simulink model "verify_Storage_Type_1_mdl"  (R2018b)
settings: Solver=ode45  StartTime=time(1)  StopTime=time(end)  MaxStep=time(2)-time(1)  RelTol=1e-3  EnableMultiTasking=on
libraries: carnot x12
settings Model: DEBUGGLOBALLEVEL=DEBUGLEVEL  DEBUGMAXTOTALWARNINGS=0  DEBUGMAXCONSECUTIVEWARNINGS=0  DEBUGWRITETOFILE=0  DEBUGFILENAME='error.txt'  Creator=drhf  LastModifiedBy=P41573
settings DataIOCC: SaveFormat=Array  SignalLoggingSaveFormat=ModelDataLogs
settings OptimizationCC: ExpressionDepthLimit=2147483647  LifeSpan=inf
settings DebuggingCC: UnderspecifiedInitializationDetection=Classic  MergeDetectMultiDrivingBlocksExec=none  SolverPrmCheckMsg=warning  FcnCallInpInsideContextMsg=warning  StateNameClashWarn=warning  SFUnexpectedBacktrackingDiag=warning  SFNoUnconditionalDefaultTransitionDiag=warning  SFExecutionAtInitializationDiag=none
settings HardwareCC: ProdBitPerPointer=32  ProdBitPerSizeT=32  ProdBitPerPtrDiffT=32  ProdLargestAtomicFloat=None  ProdIntDivRoundTo=Undefined  ProdEndianess=Unspecified  ProdWordSize=32  ProdHWDeviceType=32-bit Generic
settings ModelReferenceCC: PropagateSignalLabelsOutOfModel=off
settings SFSimCC: SimUseLocalCustomCode=off
settings RTWCC: RTWUseLocalCustomCode=off
settings CodeAppCC: StateflowObjectComments=on
settings GRTTargetCC: TargetLangStandard=C89/C90 (ANSI)  GeneratePreprocessorConditionals=Disable all  CombineOutputUpdateFcns=off  GRTInterface=on
settings ConfigComp: CovMetricSettings=dw  CovHtmlReporting=on  CovSaveCumulativeToWorkspaceVar=on  CovSaveSingleToWorkspaceVar=on  CovExternalEMLEnable=off

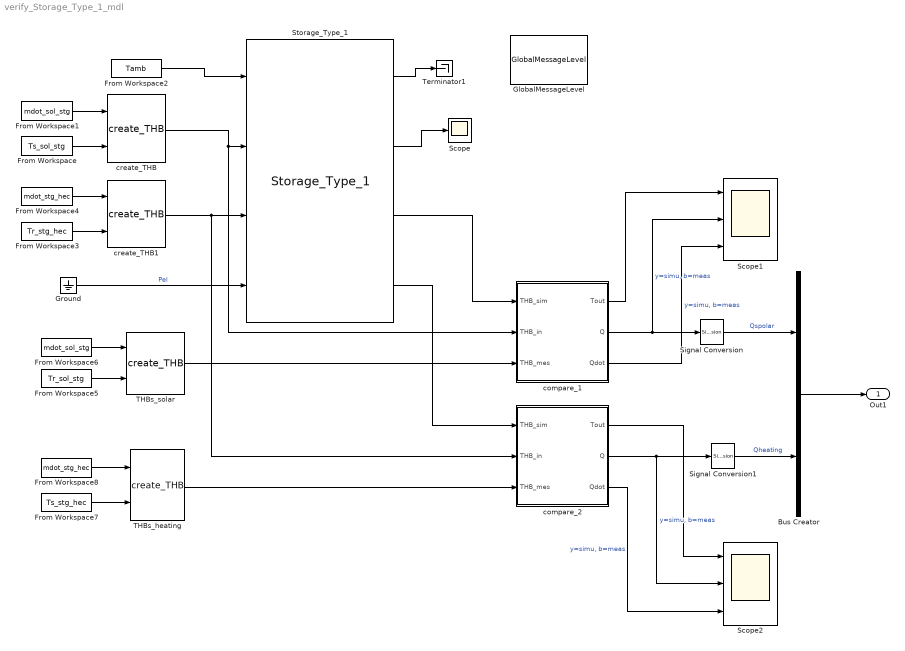
== system verify_Storage_Type_1_mdl ==
  Bus Creator : BusCreator  Inputs=2
  From Workspace : FromWorkspace  VariableName=Ts_sol_stg  SampleTime=0
  From Workspace1 : FromWorkspace  VariableName=mdot_sol_stg  SampleTime=0
  From Workspace2 : FromWorkspace  VariableName=Tamb  SampleTime=0
  From Workspace3 : FromWorkspace  VariableName=Tr_stg_hec  SampleTime=0
  From Workspace4 : FromWorkspace  VariableName=mdot_stg_hec  SampleTime=0
  From Workspace5 : FromWorkspace  VariableName=Tr_sol_stg  SampleTime=0
  From Workspace6 : FromWorkspace  VariableName=mdot_sol_stg  SampleTime=0
  From Workspace7 : FromWorkspace  VariableName=Ts_stg_hec  SampleTime=0
  From Workspace8 : FromWorkspace  VariableName=mdot_stg_hec  SampleTime=0
  GlobalMessageLevel : carnot/Toolbox/GlobalMessageLevel  GLOBALLOCAL=global  DEBUGLEVEL=DEBUGLEVEL  MAXTOTALWARNINGS=0  MAXCONSECUTIVEWARNINGS=0  WRITETOFILE=0  FILENAME='error.txt'
      settings: SourceProductName=Carnot
  Ground : Ground
  Scope : Scope
  Scope1 : Scope  NumInputPorts=3
  Scope2 : Scope  NumInputPorts=3
  Signal Conversion : SignalConversion  OverrideOpt=off
  Signal Conversion1 : SignalConversion  OverrideOpt=off
  Storage_Type_1 : carnot/Storage/Thermal/Storage_Type_1  t0=interp1(1:10, Tstg(1, 2:end), 10:-9/99:1)  hgt=0.9972  stgtype=1  tini=[21.3957 21.3967545454545 21.3978090909091 21.3988636363636 21.3999181818182 21.4009727272727 21.4020272727273 21.4030818181818 21.4041363636364 21.4051909090909 21.4062454545455 21.4073 21.4058363636364 21.4043727272727 21.4029090909091 21.4014454545455 21.3999818181818 21.3985181818182 21.3970545454545 21.3955909090909 21.3941272727273 21.3926636363636 21.3912 21.4011181818182 21.4110363636364 21.4209545454545 21.4308727272727 21.4407909090909 21.4507090909091 21.4606272727273 21.4705454545455 21.4804636363636 21.4903818181818 21.5003 21.4675909090909 21.4348818181818 21.4021727272727 21.3694636363636 21.3367545454545 21.3040454545455 21.2713363636364 21.2386272727273 21.2059181818182 21.1732090909091 21.1405 21.1688 21.1971 21.2254 21.2537 21.282 21.3103 21.3386 21.3669 21.3952 21.4235 21.4518 21.7424 22.033 22.3236 22.6142 22.9048 23.1954 23.486 23.7766 24.0672 24.3578 24.6484 25.4619090909091 26.2754181818182 27.0889272727273 27.9024363636364 28.7159454545455 29.5294545454545 30.3429636363636 31.1564727272727 31.9699818181818 32.7834909090909 33.597 33.7803636363636 33.9637272727273 34.1470909090909 34.3304545454545 34.5138181818182 34.6971818181818 34.8805454545455 35.0639090909091 35.2472727272727 35.4306363636364 35.614 35.6703 35.7266 35.7829 35.8392 35.8955 35.9518 36.0081 36.0644 36.1207 36.177 36.2333]  mpts=[3 8 13 18 23 28 33 38 43 48 53 58 63 68 73 78 83 88 93 98]  PathName='current'  FileName='Stg_verification_param.mat'  userPath=off  userParam=off  uwall=1.4  ubot=1.4  utop=1.4  axcond=1.2  volume=0.22  dia=0.53  standing=standing cylinder  nodes=100  mpoints=20  Tsensor=0.5  pipe1inlet=0.62  pipe1outlet=0  pipe1dia=0.03  pipe2inlet=0.1  pipe2outlet=1  pipe2dia=0.03  heater1start=0.6  heater1end=0.65
      settings: SourceProductName=Carnot
  THBs_heating : carnot/Source/Simple/create_THB  p=1e5  fluid=Water  mix=0  mix2=0  mix3=0  dia=0.02  hgt=0  mID=No Pressure Drop
      settings: SourceProductName=Carnot
  THBs_solar : carnot/Source/Simple/create_THB  p=1e5  fluid=Water  mix=0  mix2=0  mix3=0  dia=0.02  hgt=0  mID=No Pressure Drop
      settings: SourceProductName=Carnot
  Terminator1 : Terminator
  compare_1 : Subsystem
  compare_2 : Subsystem
  create_THB : carnot/Source/Simple/create_THB  p=1e5  fluid=Water  mix=0  mix2=0  mix3=0  dia=0.02  hgt=0  mID=No Pressure Drop
      settings: SourceProductName=Carnot
  create_THB1 : carnot/Source/Simple/create_THB  p=1e5  fluid=Water  mix=0  mix2=0  mix3=0  dia=0.02  hgt=0  mID=No Pressure Drop
      settings: SourceProductName=Carnot
  Out1 : Outport
  wires:
  From Workspace2/1 -> Storage_Type_1/1
  create_THB/1 -> Storage_Type_1/2, compare_1/2(THB_in)
  create_THB1/1 -> Storage_Type_1/3, compare_2/2(THB_in)
  Storage_Type_1/2 -> Scope/1
  Storage_Type_1/3 -> compare_1/1(THB_sim)
  Storage_Type_1/4 -> compare_2/1(THB_sim)
  Bus Creator/1 -> Out1/1
  From Workspace/1 -> create_THB/2
  From Workspace1/1 -> create_THB/1
  From Workspace4/1 -> create_THB1/1
  From Workspace3/1 -> create_THB1/2
  Storage_Type_1/1 -> Terminator1/1
  From Workspace6/1 -> THBs_solar/1
  From Workspace5/1 -> THBs_solar/2
  From Workspace8/1 -> THBs_heating/1
  From Workspace7/1 -> THBs_heating/2
  THBs_solar/1 -> compare_1/3(THB_mes)
  THBs_heating/1 -> compare_2/3(THB_mes)
  compare_1/1(Tout) -> Scope1/1
  compare_1/2(Q) -> Scope1/2, Signal Conversion/1  "y=simu, b=meas"
  compare_1/3(Qdot) -> Scope1/3  "y=simu, b=meas"
  compare_2/3(Qdot) -> Scope2/3  "y=simu, b=meas"
  compare_2/2(Q) -> Scope2/2, Signal Conversion1/1  "y=simu, b=meas"
  compare_2/1(Tout) -> Scope2/1
  Signal Conversion/1 -> Bus Creator/1  "Qspolar"
  Signal Conversion1/1 -> Bus Creator/2  "Qheating"
  Ground/1 -> Storage_Type_1/4  "Pel"

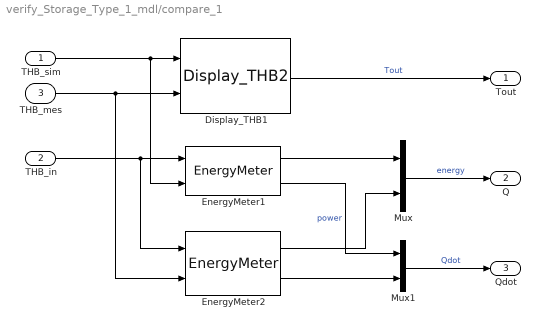
== system verify_Storage_Type_1_mdl/compare_1 ==
  THB_sim : Inport
  THB_in : Inport  Port=2
  THB_mes : Inport  Port=3
  Display_THB1 : carnot/Outputs/Display_THB2  t=on  m=off  p=off  id=off  mix=off  d=off
      settings: SourceProductName=Carnot
  EnergyMeter1 : carnot/Control/EnergyMeter
      settings: SourceProductName=Carnot
  EnergyMeter2 : carnot/Control/EnergyMeter
      settings: SourceProductName=Carnot
  Mux : Mux  Inputs=2
  Mux1 : Mux  Inputs=2
  Tout : Outport
  Q : Outport  Port=2
  Qdot : Outport  Port=3
  wires:
  THB_sim/1 -> EnergyMeter1/2, Display_THB1/1
  THB_mes/1 -> EnergyMeter2/2, Display_THB1/2
  EnergyMeter1/1 -> Mux/1
  Display_THB1/1 -> Tout/1  "Tout"
  Mux/1 -> Q/1  "energy"
  EnergyMeter1/2 -> Mux1/1  "power"
  Mux1/1 -> Qdot/1  "Qdot"
  THB_in/1 -> EnergyMeter2/1, EnergyMeter1/1
  EnergyMeter2/1 -> Mux/2
  EnergyMeter2/2 -> Mux1/2

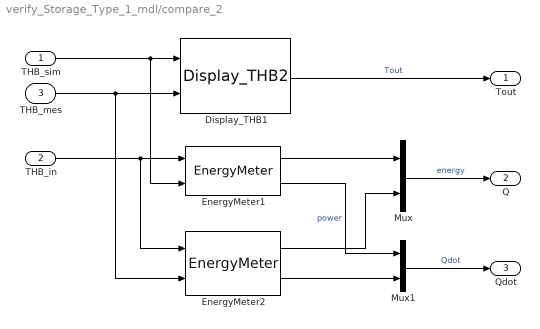
== system verify_Storage_Type_1_mdl/compare_2 ==
  THB_sim : Inport
  THB_in : Inport  Port=2
  THB_mes : Inport  Port=3
  Display_THB1 : carnot/Outputs/Display_THB2  t=on  m=off  p=off  id=off  mix=off  d=off
      settings: SourceProductName=Carnot
  EnergyMeter1 : carnot/Control/EnergyMeter
      settings: SourceProductName=Carnot
  EnergyMeter2 : carnot/Control/EnergyMeter
      settings: SourceProductName=Carnot
  Mux : Mux  Inputs=2
  Mux1 : Mux  Inputs=2
  Tout : Outport
  Q : Outport  Port=2
  Qdot : Outport  Port=3
  wires:
  EnergyMeter2/2 -> Mux1/2
  EnergyMeter2/1 -> Mux/2
  THB_in/1 -> EnergyMeter1/1, EnergyMeter2/1
  Mux1/1 -> Qdot/1  "Qdot"
  EnergyMeter1/2 -> Mux1/1  "power"
  Mux/1 -> Q/1  "energy"
  Display_THB1/1 -> Tout/1  "Tout"
  EnergyMeter1/1 -> Mux/1
  THB_mes/1 -> Display_THB1/2, EnergyMeter2/2
  THB_sim/1 -> Display_THB1/1, EnergyMeter1/2
